simulink model "Simulation_GSM_out"  (R2017b)
settings: Solver=ode15s  StartTime=0.0  StopTime=14  MaxStep=1e-3  RelTol=1e-5  AbsTol=1e-4  EnableMultiTasking=on
Description:
  | Testdatei zur Verifikation des Modells GSM mit Propeller
settings Model: Creator=wke  LastModifiedBy=Alexander Aschauer
settings DataIOCC: LimitDataPoints=on  SaveFormat=Array  SignalLoggingSaveFormat=ModelDataLogs
settings OptimizationCC: ExpressionDepthLimit=2147483647  InitFltsAndDblsToZero=on  LifeSpan=inf
settings DebuggingCC: SaveWithParameterizedLinksMsg=none  UnderspecifiedInitializationDetection=Classic  MergeDetectMultiDrivingBlocksExec=none  SolverPrmCheckMsg=warning  FcnCallInpInsideContextMsg=warning  StateNameClashWarn=warning  SFUnexpectedBacktrackingDiag=warning  SFNoUnconditionalDefaultTransitionDiag=warning  SFExecutionAtInitializationDiag=none
settings HardwareCC: ProdBitPerPointer=32  ProdBitPerSizeT=32  ProdBitPerPtrDiffT=32  ProdLargestAtomicFloat=None  ProdIntDivRoundTo=Undefined  ProdEndianess=Unspecified  ProdWordSize=32  ProdHWDeviceType=32-bit Generic
settings ModelReferenceCC: PropagateSignalLabelsOutOfModel=off
settings CodeAppCC: StateflowObjectComments=on
settings GRTTargetCC: TargetLangStandard=C89/C90 (ANSI)  GeneratePreprocessorConditionals=Disable all  CombineOutputUpdateFcns=off  GRTInterface=on
settings ConfigComp: CovMetricSettings=dw  CovHtmlReporting=on  CovSaveCumulativeToWorkspaceVar=on  CovSaveSingleToWorkspaceVar=on  CovExternalEMLEnable=off  CovSFcnEnable=off

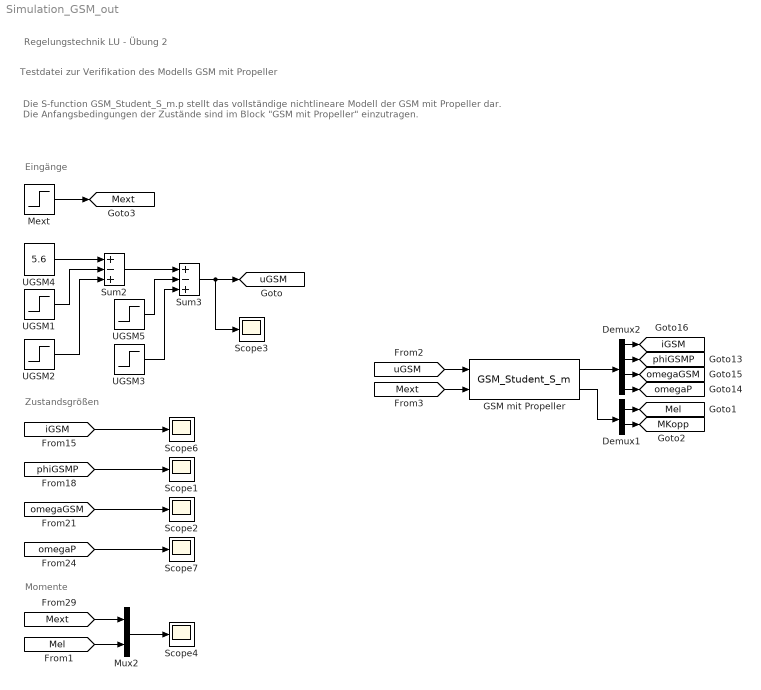
== system Simulation_GSM_out ==
  note: Eingänge
  note: Zustandsgrößen
  note: Momente
  note: Testdatei zur Verifikation des Modells GSM mit Propeller
  note: Die S-function GSM_Student_S_m.p stellt das vollständige nichtlineare Modell
      | der GSM mit Propeller dar. Die Anfangsbedingungen der Zustände sind im Block
      | "GSM mit Propeller" einzutragen.
  note: Regelungstechnik LU - Übung 2
  Demux1 : Demux  Outputs=2
  Demux2 : Demux
  GSM mit Propeller : M-S-Function  FunctionName=GSM_Student_S_m  Parameters=iGSM_0,phiGSMP_0,omegaGSM_0,omegaP_0  mask{iGSM_0=0, phiGSMP_0=0, omegaGSM_0=0, omegaP_0=0}
      mask prompts: iGSM_0 "Anfangsbedingung iGSM"; phiGSMP_0 "Anfangsbedingung phiGSMP"; omegaGSM_0 "Anfangsbedingung omegaGSM"; omegaP_0 "Anfangsbedingung omegaP"
  Mext : Step  Time=11  After=0.25  SampleTime=0
  Mux2 : Mux  Inputs=2
  Scope{1..4,6..7} (6 alike) : Scope
  Sum2 : Sum  Inputs=+-+
  Sum3 : Sum  Inputs=+-+
  UGSM1 : Step  Time=2  SampleTime=0
  UGSM2 : Step  Time=5  SampleTime=0
  UGSM3 : Step  Time=13  After=2  SampleTime=0
  UGSM4 : Constant  Value=5.6
  UGSM5 : Step  Time=8  After=2  SampleTime=0
  tag scope: MKopp=global, Mel=global, Mext=global, iGSM=global, omegaGSM=global, omegaP=global, phiGSMP=global, uGSM=global
  wires:
  [uGSM] -> GSM mit Propeller/1
  [Mext] -> GSM mit Propeller/2
  Demux2/1 -> [iGSM]
  Demux2/2 -> [phiGSMP]
  Demux2/3 -> [omegaGSM]
  Demux2/4 -> [omegaP]
  GSM mit Propeller/1 -> Demux2/1
  GSM mit Propeller/2 -> Demux1/1
  Demux1/1 -> [Mel]
  Demux1/2 -> [MKopp]
  Mext/1 -> [Mext]
  UGSM4/1 -> Sum2/1
  UGSM1/1 -> Sum2/2
  Sum2/1 -> Sum3/1
  Sum3/1 -> [uGSM], Scope3/1
  UGSM2/1 -> Sum2/3
  UGSM5/1 -> Sum3/2
  UGSM3/1 -> Sum3/3
  Mux2/1 -> Scope4/1
  [iGSM] -> Scope6/1
  [phiGSMP] -> Scope1/1
  [omegaGSM] -> Scope2/1
  [omegaP] -> Scope7/1
  [Mext] -> Mux2/1
  [Mel] -> Mux2/2
